simulink library "MyDesignedModel"  (R2019b)
settings: Solver=VariableStepAuto  StartTime=0.0  StopTime=10.0  RelTol=1e-3
libraries: powerlib_meascontrol x1
settings Model: Creator=YJR  LastModifiedBy=YJR

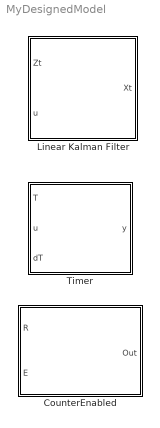
== system MyDesignedModel ==
  CounterEnabled : Subsystem  mask(CounterEnabled){}
      mask help: Count the number of square waves.
      mask Display: disp('CounterEnabled')
  Linear Kalman Filter : Subsystem  mask(Linear Kalman Filter){X0=0, P0=0, A=0, B=0, Ra=0, Qa=0, w=0}
      mask help: Linear Kalman filter
      mask Display: disp('Kalman Filter')
  Timer : Subsystem  mask(Time Count){}
      mask help: The timer starts when it is triggered, and it is output after a set time. You can set the duration and time step.
      mask Display: disp('Timer')

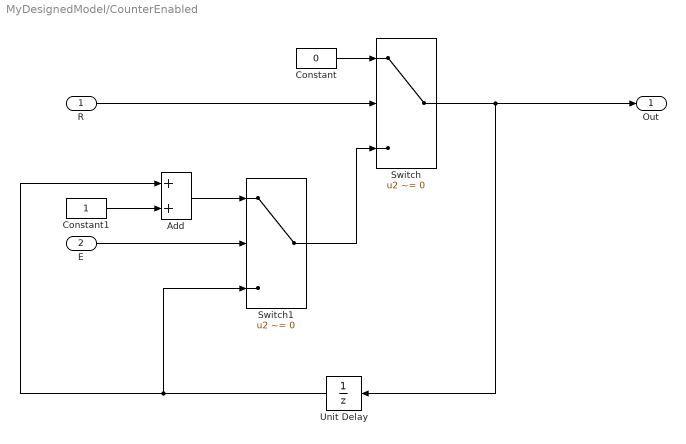
== system MyDesignedModel/CounterEnabled ==
  R : Inport
  E : Inport  Port=2
  Add : Sum
  Constant : Constant  Value=0
  Constant1 : Constant
  Switch : Switch  Criteria=u2 ~= 0
  Switch1 : Switch  Criteria=u2 ~= 0
  Unit Delay : UnitDelay  SampleTime=-1  HasFrameUpgradeWarning=on
  Out : Outport
  wires:
  Constant/1 -> Switch/1
  Switch1/1 -> Switch/3
  Switch/1 -> Out/1, Unit Delay/1
  Add/1 -> Switch1/1
  R/1 -> Switch/2
  E/1 -> Switch1/2
  Unit Delay/1 -> Switch1/3, Add/1
  Constant1/1 -> Add/2

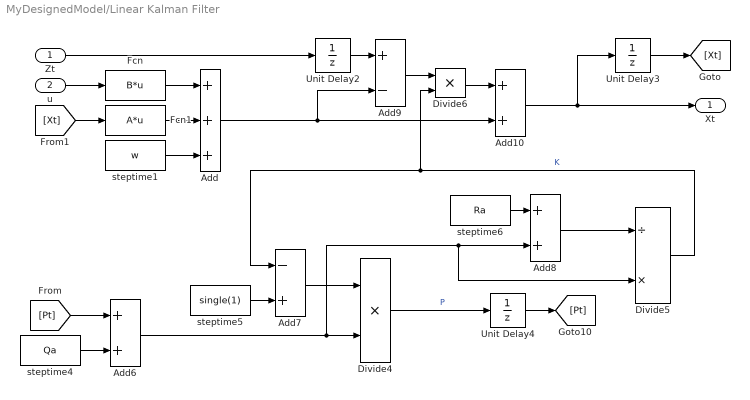
== system MyDesignedModel/Linear Kalman Filter ==
  Zt : Inport
  u : Inport  Port=2
  Add : Sum  Inputs=+++
  Add10 : Sum
  Add6 : Sum
  Add7 : Sum  Inputs=-+
  Add8 : Sum
  Add9 : Sum  Inputs=+-
  Divide4 : Product  Inputs=**
  Divide5 : Product  Inputs=/*
  Divide6 : Product  Inputs=**
  Fcn : Fcn  Expr=B*u
  Fcn1 : Fcn  Expr=A*u
  Unit Delay2 : UnitDelay  SampleTime=-1  HasFrameUpgradeWarning=on
  Unit Delay3 : UnitDelay  InitialCondition=X0  SampleTime=-1  HasFrameUpgradeWarning=on
  Unit Delay4 : UnitDelay  InitialCondition=P0  SampleTime=-1  HasFrameUpgradeWarning=on
  steptime1 : Constant  Value=w
  steptime4 : Constant  Value=Qa
  steptime5 : Constant  Value=single(1)
  steptime6 : Constant  Value=Ra
  Xt : Outport
  wires:
  [Xt] -> Fcn1/1
  Add10/1 -> Xt/1, Unit Delay3/1
  Add9/1 -> Divide6/1
  steptime5/1 -> Add7/2
  Add8/1 -> Divide5/1
  Unit Delay3/1 -> [Xt]
  Divide5/1 -> Add7/1, Divide6/2  "K"
  Add6/1 -> Divide5/2, Add8/2, Divide4/2
  Divide6/1 -> Add10/1
  Fcn1/1 -> Add/2
  steptime1/1 -> Add/3
  Zt/1 -> Unit Delay2/1
  Unit Delay2/1 -> Add9/1
  Divide4/1 -> Unit Delay4/1  "P"
  steptime4/1 -> Add6/2
  Add7/1 -> Divide4/1
  Unit Delay4/1 -> [Pt]
  u/1 -> Fcn/1
  steptime6/1 -> Add8/1
  Add/1 -> Add9/2, Add10/2
  Fcn/1 -> Add/1
  [Pt] -> Add6/1

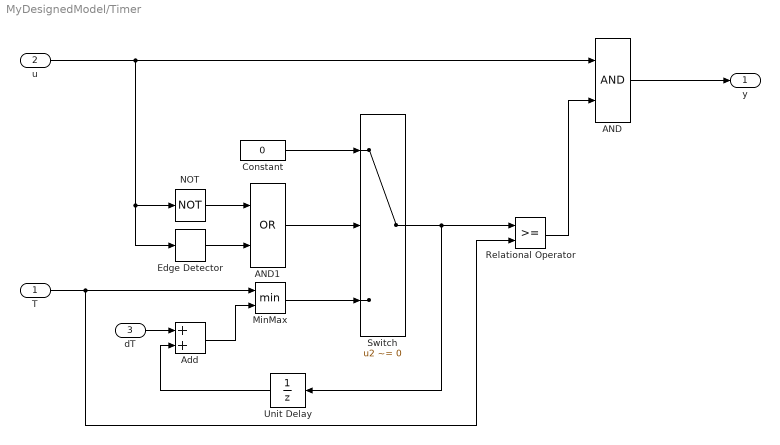
== system MyDesignedModel/Timer ==
  T : Inport
  u : Inport  Port=2
  dT : Inport  Port=3
  AND : Logic  AllPortsSameDT=off  OutDataTypeStr=boolean
  AND1 : Logic  Operator=OR  AllPortsSameDT=off  OutDataTypeStr=boolean
  Add : Sum
  Constant : Constant  Value=0
  Edge Detector : powerlib_meascontrol/Logic/Edge Detector  model=Rising  ic=0  Ts=-1
      settings: SourceProductName=Simscape Electrical  SourceProductBaseCode=PS
  MinMax : MinMax  Inputs=2
  NOT : Logic  Operator=NOT  AllPortsSameDT=off  OutDataTypeStr=boolean
  Relational Operator : RelationalOperator  OutDataTypeStr=boolean  RndMeth=Simplest
  Switch : Switch  Criteria=u2 ~= 0
  Unit Delay : UnitDelay  SampleTime=-1  HasFrameUpgradeWarning=on
  y : Outport
  wires:
  Edge Detector/1 -> AND1/2
  u/1 -> Edge Detector/1, NOT/1, AND/1
  AND/1 -> y/1
  Unit Delay/1 -> Add/2
  Add/1 -> MinMax/2
  dT/1 -> Add/1
  Switch/1 -> Relational Operator/1, Unit Delay/1
  NOT/1 -> AND1/1
  T/1 -> MinMax/1, Relational Operator/2
  Constant/1 -> Switch/1
  AND1/1 -> Switch/2
  MinMax/1 -> Switch/3
  Relational Operator/1 -> AND/2
